simulink model "ex_03_model_plot"  (R2014a)
settings: Solver=ode45  StartTime=0.0  StopTime=2  RelTol=1e-3
undefined symbols (not defined in the file or in its folder): G, x, y, z
settings Model: Creator=Nino  LastModifiedBy=Nino

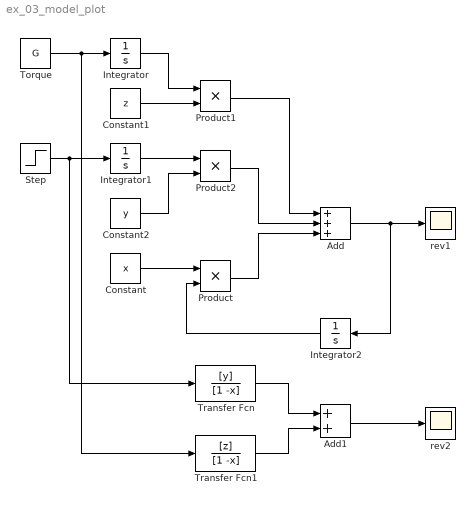
== system ex_03_model_plot ==
  Add : Sum  Inputs=+++
  Add1 : Sum
  Constant : Constant  Value=x
  Constant1 : Constant  Value=z
  Constant2 : Constant  Value=y
  Integrator : Integrator
  Integrator1 : Integrator
  Integrator2 : Integrator
  Product : Product
  Product1 : Product
  Product2 : Product
  Step : Step  After=10  SampleTime=0
  Torque : Constant  Value=G
  Transfer Fcn : TransferFcn  Numerator=[y]  Denominator=[1 -x]
  Transfer Fcn1 : TransferFcn  Numerator=[z]  Denominator=[1 -x]
  rev1 : Scope
      settings: SaveName=Rev1  SampleInput=on  SampleTime=0.01
  rev2 : Scope
      settings: SaveName=Rev2
  wires:
  Integrator2/1 -> Product/2
  Constant/1 -> Product/1
  Product/1 -> Add/3
  Add/1 -> rev1/1, Integrator2/1
  Integrator1/1 -> Product2/1
  Constant2/1 -> Product2/2
  Product2/1 -> Add/2
  Constant1/1 -> Product1/2
  Integrator/1 -> Product1/1
  Product1/1 -> Add/1
  Torque/1 -> Transfer Fcn1/1, Integrator/1
  Step/1 -> Transfer Fcn/1, Integrator1/1
  Transfer Fcn/1 -> Add1/1
  Transfer Fcn1/1 -> Add1/2
  Add1/1 -> rev2/1
